simulink library "UAVdesign_net"  (Simulink 7.7)
settings: Solver=ode45  SolverMode=SingleTasking  StartTime=0.0  StopTime=10.0  RelTol=1e-3
undefined symbols (not defined in the file or in its folder): alpha_IERA_IELA_IELA, R_IERA_RA_RA
libraries: UAVdesign_net x75, simulink x13
(part 4 of 8)

== system UAVdesign_net/Subsystem Models/Helicopter Rotor/IERA to IELA ==
  T_IELA_IERA : Inport
  FM_I_IERA : Inport  Port=2
  FM_A_IERA : Inport  Port=3
  d_IERA : Inport  Port=4
  1D : Reshape
  Demux : Demux  Outputs=[6 6 3]
  Demux1 : Demux  Outputs=2
  Demux2 : Demux  Outputs=2
  Product : Product  Multiplication=Matrix(*)  RndMeth=Zero
  Signal Specification{,1..4} (5 alike) : SignalSpecification  Dimensions=3
  Vector Concatenate : Concatenate  NumInputs=5  Mode=Multidimensional array  ConcatenateDimension=2
  FM_I_IELA : Outport
  FM_A_IELA : Outport  Port=2
  d_IELA : Outport  Port=3
  wires:
  FM_A_IERA/1 -> Demux2/1
  Demux2/2 -> Signal Specification3/1
  Demux2/1 -> Signal Specification2/1
  Demux1/1 -> Signal Specification/1
  Demux1/2 -> Signal Specification1/1
  FM_I_IERA/1 -> Demux1/1
  d_IERA/1 -> Signal Specification4/1
  Demux/3 -> d_IELA/1
  Demux/2 -> FM_A_IELA/1
  Demux/1 -> FM_I_IELA/1
  1D/1 -> Demux/1
  Product/1 -> 1D/1
  Vector Concatenate/1 -> Product/2
  T_IELA_IERA/1 -> Product/1
  Signal Specification/1 -> Vector Concatenate/1
  Signal Specification1/1 -> Vector Concatenate/2
  Signal Specification2/1 -> Vector Concatenate/3
  Signal Specification3/1 -> Vector Concatenate/4
  Signal Specification4/1 -> Vector Concatenate/5

== system UAVdesign_net/Subsystem Models/Helicopter Rotor/Rotor Model (IERA) ==
  Parameters : Inport  OutDataTypeStr=Bus: RotorParameters
  Environment : Inport  Port=2  OutDataTypeStr=Bus: Environment
  V_I : Inport  Port=3  PortDimensions=3
  omega_I : Inport  Port=4  PortDimensions=3
  V_dot_I : Inport  Port=5  PortDimensions=3
  omega_dot_I : Inport  Port=6  PortDimensions=3
  V_A : Inport  Port=7  PortDimensions=3
  omega_A : Inport  Port=8  PortDimensions=3
  omega_rotor : Inport  Port=9  PortDimensions=1
  omega_dot_rotor : Inport  Port=10  PortDimensions=1
  controls : Inport  Port=11  PortDimensions=3
  flap : Inport  Port=12  PortDimensions=3
  bt (k-1) : Inport  Port=13  PortDimensions=1
  eps0 (k-1) : Inport  Port=14  PortDimensions=1
  Ch Sign Lift : Gain  Gain=[-1 1]
  IERA to WM : Subsystem
      mask Display:
      | port_label('input', 1, 'T_{WM-IERA}', 'texmode', 'on')
      | port_label('input', 2, 'V_{I|IERA}', 'texmode', 'on')
      | port_label('input', 3, '\omega_{I|IERA}', 'texmode', 'on')
      | port_label('input', 4, 'V^\bullet_{I|IERA}', 'texmode', 'on')
      | port_label('input', 5, '\omega^\bullet_{I|IERA}', 'texmode', 'on')
      | port_label('input', 6, 'V_{A|IERA}', 'texmode', 'on')
      | port_label('input', 7, '\omega_{A|IERA}', 'texmode', 'on')
      | port_label('input', 8, 'controls_{IERA}', 'texmode', 'on')
      | port_label('input', 9, 'flap_{IERA}', 'texmode', 'on')
      | 
      | port_label('output', 1, 'V_{I|WM}', 'texmode', 'on')
      | port_label('output', 2, '\omega_{I|WM}', 'texmode', 'on')
      | port_label('output', 3, 'V^\bullet_{I|WM}', 'texmode', 'on')
      | port_label('output', 4, '\omega^\bullet_{I|WM}', 'texmode', 'on')
      | port_label('output', 5, 'V_{A|WM}', 'texmode', 'on')
      | port_label('output', 6, '\omega_{A|WM}', 'texmode', 'on')
      | port_label('output', 7, 'controls_{WM}', 'texmode', 'on')
      | port_label('output', 8, 'flap_{WM}', 'texmode', 'on')
  Rotor Flapping : Subsystem
      mask Display:
      | port_label('input', 1, 'Parameters', 'texmode', 'on')
      | port_label('input', 2, 'Environment', 'texmode', 'on')
      | port_label('input', 3, 'V_{I|WM}', 'texmode', 'on')
      | port_label('input', 4, '\omega_{I|WM}', 'texmode', 'on')
      | port_label('input', 5, 'V^\bullet_{I|WM}', 'texmode', 'on')
      | port_label('input', 6, '\omega^\bullet_{I|WM}', 'texmode', 'on')
      | port_label('input', 7, 'V_{A|WM}', 'texmode', 'on')
      | port_label('input', 8, '\omega_{A|WM}', 'texmode', 'on')
      | port_label('input', 9, 'flap_{WM}', 'texmode', 'on')
      | port_label('input', 10, 'cz', 'texmode', 'on')
      | port_label('input', 11, 'controls_{WM}', 'texmode', 'on')
      | port_label('input', 12, '\Omega_{rotor}', 'texmode', 'on')
      | 
      | port_label('output', 1, 'flap^\bullet_{WM}', 'texmode', 'on')
      | port_label('output', 2, 'flap-static_{WM}', 'texmode', 'on')
  Rotor Forces and Moments : Subsystem
      mask Display:
      | port_label('input', 1, 'Parameters', 'texmode', 'on')
      | port_label('input', 2, 'Environment', 'texmode', 'on')
      | port_label('input', 3, 'V_{A|WM}', 'texmode', 'on')
      | port_label('input', 4, '\omega_{A|WM}', 'texmode', 'on')
      | port_label('input', 5, '\omega^\bullet_{I|WM}', 'texmode', 'on')
      | port_label('input', 6, 'flap_{WM}', 'texmode', 'on')
      | port_label('input', 7, 'cz', 'texmode', 'on')
      | port_label('input', 8, 'controls_{WM}', 'texmode', 'on')
      | port_label('input', 9, '\Omega_{rotor}', 'texmode', 'on')
      | port_label('input', 10, '\Omega^\bullet_{rotor}', 'texmode', 'on')
      | 
      | port_label('output', 1, 'FM_{A}', 'texmode', 'on')
      | port_label('output', 2, 'FM_{I}', 'texmode', 'on')
  Rotor Self-Influence : Subsystem
      mask Display:
      | port_label('input', 1, 'Parameters', 'texmode', 'on')
      | port_label('input', 2, 'Environment', 'texmode', 'on')
      | port_label('input', 3, 'V_{A|IERA}', 'texmode', 'on')
      | port_label('input', 4, '\omega_{A|IERA}', 'texmode', 'on')
      | port_label('input', 5, 'FM_{A|IERA}', 'texmode', 'on')
      | 
      | port_label('output', 1, 'd_{k|IERA}', 'texmode', 'on')
  Rotor Wash Iteration : Subsystem
      mask Display:
      | port_label('input', 1, 'Parameters', 'texmode', 'on')
      | port_label('input', 2, 'V_{I|WM}', 'texmode', 'on')
      | port_label('input', 3, 'V_{A k-1|WM}', 'texmode', 'on')
      | port_label('input', 4, '\omega_{A|WM}', 'texmode', 'on')
      | port_label('input', 5, 'bt_{k-1}', 'texmode', 'on')
      | port_label('input', 6, 'eps0_{k-1}', 'texmode', 'on')
      | port_label('input', 7, 'controls_{WM}', 'texmode', 'on')
      | port_label('input', 8, '\Omega_{rotor}', 'texmode', 'on')
      | 
      | port_label('output', 1, 'V_{A k|WM}', 'texmode', 'on')
      | port_label('output', 2, 'cz_{k|WM}', 'texmode', 'on')
      | port_label('output', 3, 'bt_{k}', 'texmode', 'on')
      | port_label('output', 4, 'eps_{k}', 'texmode', 'on')
  T Q : Selector  InputPortWidth=6  IndexOptions=Index vector (dialog)  Indices=[3 6]  OutputSizes=1
  WM to IERA : Subsystem
      mask Display:
      | port_label('input', 1, 'T_{IERA-WM}', 'texmode', 'on')
      | port_label('input', 2, 'FM_{A|WM}', 'texmode', 'on')
      | port_label('input', 3, 'FM_{I|WM}', 'texmode', 'on')
      | port_label('input', 4, 'V_{A k|WM}', 'texmode', 'on')
      | port_label('input', 5, 'flap^\bullet_{WM}', 'texmode', 'on')
      | port_label('input', 6, 'flap_{WM}', 'texmode', 'on')
      | 
      | port_label('output', 1, 'FM_{A|IERA}', 'texmode', 'on')
      | port_label('output', 2, 'FM_{I|IERA}', 'texmode', 'on')
      | port_label('output', 3, 'V_{A k|IERA}', 'texmode', 'on')
      | port_label('output', 4, 'flap^\bullet_{IERA}', 'texmode', 'on')
      | port_label('output', 5, 'flap_{IERA}', 'texmode', 'on')
  Wind-Mast Orientation : Subsystem
      mask Display:
      | port_label('input', 1, 'V_{A|IERA}', 'texmode', 'on')
      | port_label('output', 1, 'T_{WM-IERA}', 'texmode', 'on')
      | port_label('output', 2, 'T_{IERA-WM}', 'texmode', 'on')
  FM_I : Outport  PortDimensions=6
  FM_A : Outport  Port=2  PortDimensions=6
  d (k) : Outport  Port=3  PortDimensions=3
  flap_dot : Outport  Port=4  PortDimensions=3
  flap (k) : Outport  Port=5  PortDimensions=3
  bt (k) : Outport  Port=6  PortDimensions=1
  eps0 (k) : Outport  Port=7  PortDimensions=1
  TQ : Outport  Port=8  PortDimensions=2
  wires:
  eps0 (k-1)/1 -> Rotor Wash Iteration/6(eps0 (k-1))
  bt (k-1)/1 -> Rotor Wash Iteration/5(bt (k-1))
  Rotor Wash Iteration/4(eps0 (k)) -> eps0 (k)/1
  Rotor Wash Iteration/3(bt (k)) -> bt (k)/1
  WM to IERA/5(flap_IERA) -> flap (k)/1
  WM to IERA/4(flap_dot_IERA) -> flap_dot/1
  WM to IERA/1(FM_A_IERA) -> FM_A/1, Rotor Self-Influence/5(FM_A)
  WM to IERA/2(FM_I_IERA) -> FM_I/1
  Rotor Flapping/2(flap_static) -> WM to IERA/6(flap_WM)
  Rotor Flapping/1(flap_dot) -> WM to IERA/5(flap_dot_WM)
  Rotor Forces and Moments/2(FM_I) -> WM to IERA/3(FM_I_WM)
  Rotor Forces and Moments/1(FM_A) -> WM to IERA/2(FM_A_WM), T Q/1
  Wind-Mast Orientation/2(T_IERA_WM) -> WM to IERA/1(T_IERA_WM)
  omega_dot_rotor/1 -> Rotor Forces and Moments/10(omega_dot_rotor)
  omega_rotor/1 -> Rotor Forces and Moments/9(omega_rotor), Rotor Wash Iteration/8(omega_rotor), Rotor Flapping/12(omega)
  IERA to WM/8(flap_WM) -> Rotor Forces and Moments/6(flap), Rotor Flapping/9(flap)
  IERA to WM/7(controls_WM) -> Rotor Wash Iteration/7(controls), Rotor Flapping/11(controls), Rotor Forces and Moments/8(controls)
  Rotor Wash Iteration/2(cz (k)) -> Rotor Flapping/10(cz), Rotor Forces and Moments/7(cz)
  IERA to WM/1(V_I_WM) -> Rotor Flapping/3(V_I), Rotor Wash Iteration/2(V_I)
  IERA to WM/2(omega_I_WM) -> Rotor Flapping/4(omega_I)
  IERA to WM/3(V_dot_I_WM) -> Rotor Flapping/5(V_dot_I)
  IERA to WM/4(omega_dot_I_WM) -> Rotor Flapping/6(omega_dot_I), Rotor Forces and Moments/5(omega_dot_I)
  IERA to WM/6(omega_A_WM) -> Rotor Wash Iteration/4(omega_A), Rotor Flapping/8(omega_A), Rotor Forces and Moments/4(omega_A)
  Environment/1 -> Rotor Forces and Moments/2(Environment), Rotor Flapping/2(Environment), Rotor Self-Influence/2(Environment)
  Parameters/1 -> Rotor Forces and Moments/1(Parameters), Rotor Flapping/1(Parameters), Rotor Wash Iteration/1(Parameters), Rotor Self-Influence/1(Parameters)
  flap/1 -> IERA to WM/9(flap_IERA)
  omega_I/1 -> IERA to WM/3(omega_I_IERA)
  controls/1 -> IERA to WM/8(controls_IERA)
  Wind-Mast Orientation/1(T_WM_IERA) -> IERA to WM/1(T_WM_IERA)
  omega_A/1 -> IERA to WM/7(omega_A_IERA), Rotor Self-Influence/4(omega_A)
  V_A/1 -> Wind-Mast Orientation/1(V_A), IERA to WM/6(V_A_IERA)
  omega_dot_I/1 -> IERA to WM/5(omega_dot_I_IERA)
  V_dot_I/1 -> IERA to WM/4(V_dot_I_IERA)
  V_I/1 -> IERA to WM/2(V_I_IERA)
  IERA to WM/5(V_A_WM) -> Rotor Wash Iteration/3(V_A (k-1))
  Rotor Wash Iteration/1(V_A (k)) -> Rotor Forces and Moments/3(V_A), Rotor Flapping/7(V_A), WM to IERA/4(d_WM)
  WM to IERA/3(d_IERA) -> Rotor Self-Influence/3(V_A)
  Rotor Self-Influence/1(d (k)) -> d (k)/1
  T Q/1 -> Ch Sign Lift/1
  Ch Sign Lift/1 -> TQ/1

== system UAVdesign_net/Subsystem Models/Helicopter Rotor/Transpose ==
  In : Inport
  Permute Dimensions : PermuteDimensions
  Out : Outport
  wires:
  In/1 -> Permute Dimensions/1
  Permute Dimensions/1 -> Out/1

== system UAVdesign_net/Subsystem Models/Propeller/CG to IELA ==
  R_IELA-B|B : Inport
  V_B-E|B : Inport  Port=2
  omega_B_E|B : Inport  Port=3
  3x3 Cross Product : UAVdesign_net/Utilities/Math/3x3 Cross Product  SystemSampleTime=-1
  Sum : Sum  Inputs=++|
  V_IELA-E|IELA : Outport
  omega_IELA-E|IELA : Outport  Port=2
  wires:
  omega_B_E|B/1 -> 3x3 Cross Product/1, omega_IELA-E|IELA/1
  R_IELA-B|B/1 -> 3x3 Cross Product/2
  3x3 Cross Product/1 -> Sum/2
  V_B-E|B/1 -> Sum/1
  Sum/1 -> V_IELA-E|IELA/1

== system UAVdesign_net/Subsystem Models/Propeller/Direction of Rotation ==
  Parameters : Inport
  V_B-E|B_in : Inport  Port=2
  omega_B_E|B_in : Inport  Port=3
  V_W|B_in : Inport  Port=4
  omega_W|B_in : Inport  Port=5
  d|B_in : Inport  Port=6
  Bus Selector : BusSelector  OutputSignals=azsign
  Constant : Constant
  Mux : Mux  Inputs=3
  Mux1 : Mux  Inputs=3
  Product{,1..4} (5 alike) : Product  RndMeth=Zero
  Unary Minus : UnaryMinus
  V_B-E|B : Outport
  omega_B_E|B : Outport  Port=2
  V_W|B : Outport  Port=3
  omega_W|B : Outport  Port=4
  d|B : Outport  Port=5
  wires:
  Parameters/1 -> Bus Selector/1
  Bus Selector/1 -> Unary Minus/1  "<azsign>"
  Unary Minus/1 -> Mux/1, Mux/3, Mux1/2
  Constant/1 -> Mux/2, Mux1/1, Mux1/3
  V_B-E|B_in/1 -> Product/2
  Product/1 -> V_B-E|B/1
  Mux1/1 -> Product/1, Product3/1, Product4/1
  Mux/1 -> Product2/1, Product1/1
  omega_B_E|B_in/1 -> Product2/2
  Product2/1 -> omega_B_E|B/1
  Product3/1 -> V_W|B/1
  Product1/1 -> omega_W|B/1
  Product4/1 -> d|B/1
  V_W|B_in/1 -> Product3/2
  omega_W|B_in/1 -> Product1/2
  d|B_in/1 -> Product4/2

== system UAVdesign_net/Subsystem Models/Propeller/Direction of Rotation 2 ==
  Parameters : Inport
  FM_IELA_in : Inport  Port=2
  d_IELA_in : Inport  Port=3
  Bus Selector : BusSelector  OutputSignals=azsign
  Constant : Constant
  Mux : Mux  Inputs=6
  Mux1 : Mux  Inputs=3
  Product : Product  RndMeth=Zero
  Product1 : Product  RndMeth=Zero
  Unary Minus : UnaryMinus
  FM_IELA : Outport
  d_IELA : Outport  Port=2
  wires:
  Product/1 -> FM_IELA/1
  FM_IELA_in/1 -> Product/2
  Bus Selector/1 -> Unary Minus/1  "<azsign>"
  Parameters/1 -> Bus Selector/1
  Unary Minus/1 -> Mux/2, Mux/4, Mux/6, Mux1/2
  Constant/1 -> Mux/1, Mux/3, Mux/5, Mux1/1, Mux1/3
  Mux/1 -> Product/1
  Mux1/1 -> Product1/1
  Product1/1 -> d_IELA/1
  d_IELA_in/1 -> Product1/2

== system UAVdesign_net/Subsystem Models/Propeller/IELA to CG ==
  R_IELA_B_B : Inport
  FM_IELA : Inport  Port=2
  3x3 Cross Product : UAVdesign_net/Utilities/Math/3x3 Cross Product  SystemSampleTime=-1
  Demux : Demux  Outputs=2
  Mux : Mux  Inputs=2
  Sum : Sum  Inputs=++|
  FM_B : Outport
  wires:
  FM_IELA/1 -> Demux/1
  Mux/1 -> FM_B/1
  Demux/1 -> Mux/1, 3x3 Cross Product/2
  R_IELA_B_B/1 -> 3x3 Cross Product/1
  Demux/2 -> Sum/2
  Sum/1 -> Mux/2
  3x3 Cross Product/1 -> Sum/1

== system UAVdesign_net/Subsystem Models/Propeller/IELA to IERA ==
  T_IERA_IELA : Inport
  V_I_IELA : Inport  Port=2
  omega_I_IELA : Inport  Port=3
  V_A_IELA : Inport  Port=4
  omega_A_IELA : Inport  Port=5
  1D : Reshape
  Demux : Demux
  Product : Product  Multiplication=Matrix(*)  RndMeth=Zero
  Vector Concatenate : Concatenate  NumInputs=4  Mode=Multidimensional array  ConcatenateDimension=2
  V_I_IERA : Outport
  omega_I_IERA : Outport  Port=2
  V_A_IERA : Outport  Port=3
  omega_A_IERA : Outport  Port=4
  wires:
  T_IERA_IELA/1 -> Product/1
  V_I_IELA/1 -> Vector Concatenate/1
  omega_I_IELA/1 -> Vector Concatenate/2
  Vector Concatenate/1 -> Product/2
  Product/1 -> 1D/1
  1D/1 -> Demux/1
  Demux/1 -> V_I_IERA/1
  Demux/2 -> omega_I_IERA/1
  Demux/3 -> V_A_IERA/1
  Demux/4 -> omega_A_IERA/1
  V_A_IELA/1 -> Vector Concatenate/3
  omega_A_IELA/1 -> Vector Concatenate/4

== system UAVdesign_net/Subsystem Models/Propeller/IERA to IELA ==
  T_IELA_IERA : Inport
  FM_IERA : Inport  Port=2
  d_IERA : Inport  Port=3
  1D : Reshape
  Demux : Demux  Outputs=[6 3]
  Demux1 : Demux  Outputs=2
  Product : Product  Multiplication=Matrix(*)  RndMeth=Zero
  Signal Specification : SignalSpecification  Dimensions=3
  Signal Specification1 : SignalSpecification  Dimensions=3
  Signal Specification4 : SignalSpecification  Dimensions=3
  Vector Concatenate : Concatenate  NumInputs=3  Mode=Multidimensional array  ConcatenateDimension=2
  FM_IELA : Outport
  d_IELA : Outport  Port=2
  wires:
  Signal Specification4/1 -> Vector Concatenate/3
  Signal Specification1/1 -> Vector Concatenate/2
  Signal Specification/1 -> Vector Concatenate/1
  T_IELA_IERA/1 -> Product/1
  Vector Concatenate/1 -> Product/2
  Product/1 -> 1D/1
  1D/1 -> Demux/1
  Demux/1 -> FM_IELA/1
  d_IERA/1 -> Signal Specification4/1
  FM_IERA/1 -> Demux1/1
  Demux1/2 -> Signal Specification1/1
  Demux1/1 -> Signal Specification/1
  Demux/2 -> d_IELA/1

== system UAVdesign_net/Subsystem Models/Propeller/Rotor Forces and Moments (Inertial) ==
  Parameters : Inport
  FM_A_IERA : Inport  Port=2
  omega_I : Inport  Port=3
  omega_rotor : Inport  Port=4
  torque_motor : Inport  Port=5
  Rotor Forces and Moments (IERA) : Stateflow chart  TreatAsAtomicUnit=on
  FM_total : Outport  PortDimensions=6
  wires:
  FM_A_IERA/1 -> Rotor Forces and Moments (IERA)/5(FM_A)
  omega_I/1 -> Rotor Forces and Moments (IERA)/2(omi)
  Rotor Forces and Moments (IERA)/1(FM_total) -> FM_total/1
  Parameters/1 -> Rotor Forces and Moments (IERA)/1(Parameters)
  omega_rotor/1 -> Rotor Forces and Moments (IERA)/3(omega)
  torque_motor/1 -> Rotor Forces and Moments (IERA)/4(tau_motor)

== system UAVdesign_net/Subsystem Models/Propeller/Rotor Model (IERA) ==
  Parameters : Inport
  Environment : Inport  Port=2
  V_I : Inport  Port=3  PortDimensions=3
  omega_I : Inport  Port=4  PortDimensions=3
  V_A : Inport  Port=5  PortDimensions=3
  omega_A : Inport  Port=6  PortDimensions=3
  omega_rotor : Inport  Port=7  PortDimensions=1
  controls : Inport  Port=8  PortDimensions=1
  bt (k-1) : Inport  Port=9  PortDimensions=1
  eps0 (k-1) : Inport  Port=10  PortDimensions=1
  Ch Sign Lift : Gain  Gain=[-1 1]
  IERA to WM : Subsystem
      mask Display:
      | port_label('input', 1, 'T_{WM-IERA}', 'texmode', 'on')
      | port_label('input', 2, 'V_{I|IERA}', 'texmode', 'on')
      | port_label('input', 3, '\omega_{I|IERA}', 'texmode', 'on')
      | port_label('input', 4, 'V_{A|IERA}', 'texmode', 'on')
      | port_label('input', 5, '\omega_{A|IERA}', 'texmode', 'on')
      | 
      | port_label('output', 1, 'V_{I|WM}', 'texmode', 'on')
      | port_label('output', 2, '\omega_{I|WM}', 'texmode', 'on')
      | port_label('output', 3, 'V_{A|WM}', 'texmode', 'on')
      | port_label('output', 4, '\omega_{A|WM}', 'texmode', 'on')
  Rotor Forces and Moments (Aero) : Subsystem
      mask Display:
      | port_label('input', 1, 'Parameters', 'texmode', 'on')
      | port_label('input', 2, 'Environment', 'texmode', 'on')
      | port_label('input', 3, 'V_{A|WM}', 'texmode', 'on')
      | port_label('input', 4, '\omega_{A|WM}', 'texmode', 'on')
      | port_label('input', 5, 'cz', 'texmode', 'on')
      | port_label('input', 6, 'controls_{WM}', 'texmode', 'on')
      | port_label('input', 7, '\Omega_{rotor}', 'texmode', 'on')
      | 
      | port_label('output', 1, 'FM_{A}', 'texmode', 'on')
  Rotor Self-Influence : Subsystem
      mask Display:
      | port_label('input', 1, 'Parameters', 'texmode', 'on')
      | port_label('input', 2, 'Environment', 'texmode', 'on')
      | port_label('input', 3, 'V_{A|IERA}', 'texmode', 'on')
      | port_label('input', 4, '\omega_{A|IERA}', 'texmode', 'on')
      | port_label('input', 5, 'FM_{A|IERA}', 'texmode', 'on')
      | 
      | port_label('output', 1, 'd_{k|IERA}', 'texmode', 'on')
  Rotor Wash Iteration : Subsystem
      mask Display:
      | port_label('input', 1, 'Parameters', 'texmode', 'on')
      | port_label('input', 2, 'V_{I|WM}', 'texmode', 'on')
      | port_label('input', 3, 'V_{A k-1|WM}', 'texmode', 'on')
      | port_label('input', 4, '\omega_{A|WM}', 'texmode', 'on')
      | port_label('input', 5, 'bt_{k-1}', 'texmode', 'on')
      | port_label('input', 6, 'eps0_{k-1}', 'texmode', 'on')
      | port_label('input', 7, 'controls_{WM}', 'texmode', 'on')
      | port_label('input', 8, '\Omega_{rotor}', 'texmode', 'on')
      | 
      | port_label('output', 1, 'V_{A k|WM}', 'texmode', 'on')
      | port_label('output', 2, 'cz_{k|WM}', 'texmode', 'on')
      | port_label('output', 3, 'bt_{k}', 'texmode', 'on')
      | port_label('output', 4, 'eps_{k}', 'texmode', 'on')
  T Q : Selector  InputPortWidth=6  IndexOptions=Index vector (dialog)  Indices=[3 6]  OutputSizes=1
  Terminator : Terminator
  WM to IERA : Subsystem
      mask Display:
      | port_label('input', 1, 'T_{IERA-WM}', 'texmode', 'on')
      | port_label('input', 2, 'FM_{A|WM}', 'texmode', 'on')
      | port_label('input', 3, 'V_{A k|WM}', 'texmode', 'on')
      | 
      | port_label('output', 1, 'FM_{A|IERA}', 'texmode', 'on')
      | port_label('output', 2, 'V_{A k|IERA}', 'texmode', 'on')
  Wind-Mast Orientation : Subsystem
      mask Display:
      | port_label('input', 1, 'V_{A|IERA}', 'texmode', 'on')
      | port_label('output', 1, 'T_{WM-IERA}', 'texmode', 'on')
      | port_label('output', 2, 'T_{IERA-WM}', 'texmode', 'on')
  FM_A : Outport  PortDimensions=6
  d (k) : Outport  Port=2  PortDimensions=3
  bt (k) : Outport  Port=3  PortDimensions=1
  eps0 (k) : Outport  Port=4  PortDimensions=1
  TQ : Outport  Port=5  PortDimensions=2
  wires:
  Ch Sign Lift/1 -> TQ/1
  T Q/1 -> Ch Sign Lift/1
  Rotor Self-Influence/1(d (k)) -> d (k)/1
  WM to IERA/2(d_IERA) -> Rotor Self-Influence/3(V_A)
  Rotor Wash Iteration/1(V_A (k)) -> WM to IERA/3(d_WM), Rotor Forces and Moments (Aero)/3(V_A)
  IERA to WM/3(V_A_WM) -> Rotor Wash Iteration/3(V_A (k-1))
  V_I/1 -> IERA to WM/2(V_I_IERA)
  V_A/1 -> IERA to WM/4(V_A_IERA), Wind-Mast Orientation/1(V_A)
  omega_A/1 -> Rotor Self-Influence/4(omega_A), IERA to WM/5(omega_A_IERA)
  Wind-Mast Orientation/1(T_WM_IERA) -> IERA to WM/1(T_WM_IERA)
  omega_I/1 -> IERA to WM/3(omega_I_IERA)
  Parameters/1 -> Rotor Forces and Moments (Aero)/1(Parameters), Rotor Wash Iteration/1(Parameters), Rotor Self-Influence/1(Parameters)
  Environment/1 -> Rotor Forces and Moments (Aero)/2(Environment), Rotor Self-Influence/2(Environment)
  IERA to WM/4(omega_A_WM) -> Rotor Forces and Moments (Aero)/4(omega_A), Rotor Wash Iteration/4(omega_A)
  IERA to WM/1(V_I_WM) -> Rotor Wash Iteration/2(V_I)
  Rotor Wash Iteration/2(cz (k)) -> Rotor Forces and Moments (Aero)/5(cz)
  omega_rotor/1 -> Rotor Wash Iteration/8(omega_rotor), Rotor Forces and Moments (Aero)/7(omega_rotor)
  Wind-Mast Orientation/2(T_IERA_WM) -> WM to IERA/1(T_IERA_WM)
  Rotor Forces and Moments (Aero)/1(FM_A) -> T Q/1, WM to IERA/2(FM_A_WM)
  WM to IERA/1(FM_A_IERA) -> FM_A/1, Rotor Self-Influence/5(FM_A)
  Rotor Wash Iteration/3(bt (k)) -> bt (k)/1
  Rotor Wash Iteration/4(eps0 (k)) -> eps0 (k)/1
  bt (k-1)/1 -> Rotor Wash Iteration/5(bt (k-1))
  eps0 (k-1)/1 -> Rotor Wash Iteration/6(eps0 (k-1))
  controls/1 -> Rotor Forces and Moments (Aero)/6(controls), Rotor Wash Iteration/7(controls)
  IERA to WM/2(omega_I_WM) -> Terminator/1

== system UAVdesign_net/Subsystem Models/Propeller/Transpose ==
  In : Inport
  Permute Dimensions : PermuteDimensions
  Out : Outport
  wires:
  Permute Dimensions/1 -> Out/1
  In/1 -> Permute Dimensions/1

== system UAVdesign_net/Subsystem Models/Propeller Rotation Dynamics/Direction of Rotation ==
  Parameters : Inport
  omega_B_E|B_in : Inport  Port=2
  omega_dot_B_E|B_in : Inport  Port=3
  Bus Selector : BusSelector  OutputSignals=azsign
  Constant : Constant
  Mux : Mux  Inputs=3
  Product1 : Product  RndMeth=Zero
  Product2 : Product  RndMeth=Zero
  Unary Minus : simulink/Math Operations/Unary Minus  DoSatur=off
  omega_B_E|B : Outport
  omega_dot_B_E|B : Outport  Port=2
  wires:
  Product2/1 -> omega_B_E|B/1
  omega_B_E|B_in/1 -> Product2/2
  Mux/1 -> Product2/1, Product1/1
  Constant/1 -> Mux/2
  Unary Minus/1 -> Mux/1, Mux/3
  Bus Selector/1 -> Unary Minus/1  "<azsign>"
  Parameters/1 -> Bus Selector/1
  Product1/1 -> omega_dot_B_E|B/1
  omega_dot_B_E|B_in/1 -> Product1/2

== system UAVdesign_net/Subsystem Models/Propeller Rotation Dynamics/IELA to IERA ==
  T_IERA_IELA : Inport
  omega_I_IELA : Inport  Port=2
  omega_dot_I_IELA : Inport  Port=3
  1D : Reshape
  Demux : Demux  Outputs=2
  Product : Product  Multiplication=Matrix(*)  RndMeth=Zero
  Vector Concatenate : Concatenate  Mode=Multidimensional array  ConcatenateDimension=2
  omega_I_IERA : Outport
  omega_dot_I_IERA : Outport  Port=2
  wires:
  1D/1 -> Demux/1
  Product/1 -> 1D/1
  Vector Concatenate/1 -> Product/2
  T_IERA_IELA/1 -> Product/1
  omega_I_IELA/1 -> Vector Concatenate/1
  omega_dot_I_IELA/1 -> Vector Concatenate/2
  Demux/2 -> omega_dot_I_IERA/1
  Demux/1 -> omega_I_IERA/1

== system UAVdesign_net/Subsystem Models/QuadRotor Parameters/Fuse Parameters ==
  In : Inport
  Bus Creator : BusCreator  Inputs=7  OutDataTypeStr=Bus: FuselageParameters  NonVirtualBus=on
  Demux : Demux  Outputs=17
  Vector Concatenate{,1..4} (5 alike) : Concatenate  NumInputs=3  Mode=Vector
  Parameters : Outport  OutDataTypeStr=Bus: FuselageParameters
  wires:
  Demux/1 -> Bus Creator/1  "carea"
  Bus Creator/1 -> Parameters/1
  In/1 -> Demux/1
  Demux/2 -> Bus Creator/2  "clen"
  Demux/3 -> Vector Concatenate/1
  Demux/4 -> Vector Concatenate/2
  Demux/5 -> Vector Concatenate/3
  Vector Concatenate/1 -> Bus Creator/3  "cx"
  Demux/6 -> Vector Concatenate1/1
  Demux/7 -> Vector Concatenate1/2
  Demux/8 -> Vector Concatenate1/3
  Vector Concatenate1/1 -> Bus Creator/4  "cy"
  Demux/9 -> Vector Concatenate2/1
  Demux/10 -> Vector Concatenate2/2
  Demux/11 -> Vector Concatenate2/3
  Vector Concatenate2/1 -> Bus Creator/5  "cz"
  Demux/12 -> Vector Concatenate3/1
  Demux/13 -> Vector Concatenate3/2
  Demux/14 -> Vector Concatenate3/3
  Demux/15 -> Vector Concatenate4/1
  Demux/16 -> Vector Concatenate4/2
  Demux/17 -> Vector Concatenate4/3
  Vector Concatenate3/1 -> Bus Creator/6  "cm"
  Vector Concatenate4/1 -> Bus Creator/7  "cn"

== system UAVdesign_net/Subsystem Models/QuadRotor Parameters/Motor Parameters ==
  In : Inport
  Bus Creator1 : BusCreator  Inputs=7  NonVirtualBus=on
  Data Type Conversion2 : DataTypeConversion  OutDataTypeStr=uint32  RndMeth=Nearest
  Demux1 : Demux  Outputs=7
  Parameters : Outport
  wires:
  In/1 -> Demux1/1
  Bus Creator1/1 -> Parameters/1
  Demux1/1 -> Bus Creator1/1  "R"
  Demux1/2 -> Bus Creator1/2  "L"
  Demux1/3 -> Bus Creator1/3  "Kv"
  Demux1/4 -> Bus Creator1/4  "Kt"
  Demux1/5 -> Data Type Conversion2/1
  Data Type Conversion2/1 -> Bus Creator1/5  "poles"
  Demux1/6 -> Bus Creator1/6  "In"
  Demux1/7 -> Bus Creator1/7  "Ngear"

== system UAVdesign_net/Subsystem Models/QuadRotor Parameters/Rotor Parameters ==
  In : Inport
  Bus Creator1 : BusCreator  Inputs=14  NonVirtualBus=on
  Data Type Conversion1 : DataTypeConversion  OutDataTypeStr=uint32  RndMeth=Nearest
  Data Type Conversion2 : DataTypeConversion  OutDataTypeStr=uint32  RndMeth=Nearest
  Demux1 : Demux  Outputs=16
  Gain1 : Gain  Gain=pi/180
  Gain3 : Gain  Gain=pi/180
  Vector Concatenate : Concatenate  NumInputs=3  Mode=Vector
  Parameters : Outport
  wires:
  Demux1/15 -> Bus Creator1/13  "azsign"
  Demux1/14 -> Bus Creator1/12  "mbar"
  Demux1/13 -> Bus Creator1/11  "iflap"
  Demux1/9 -> Bus Creator1/7  "btmax"
  Demux1/1 -> Bus Creator1/1  "a0"
  Bus Creator1/1 -> Parameters/1
  Demux1/4 -> Vector Concatenate/3
  Demux1/3 -> Vector Concatenate/2
  Demux1/2 -> Vector Concatenate/1
  In/1 -> Demux1/1
  Data Type Conversion1/1 -> Bus Creator1/3  "nb"
  Demux1/5 -> Data Type Conversion1/1
  Demux1/6 -> Bus Creator1/4  "radius"
  Demux1/7 -> Bus Creator1/5  "chord"
  Demux1/8 -> Bus Creator1/6  "btmin"
  Demux1/12 -> Gain3/1
  Demux1/10 -> Bus Creator1/8  "btq"
  Demux1/11 -> Gain1/1  "theta"
  Gain1/1 -> Bus Creator1/9  "theta"
  Vector Concatenate/1 -> Bus Creator1/2  "del0_2"
  Gain3/1 -> Bus Creator1/10  "twist"
  Demux1/16 -> Data Type Conversion2/1
  Data Type Conversion2/1 -> Bus Creator1/14  "flags"

== system UAVdesign_net/Subsystem Models/Wing/CG to IELA ==
  R_IELA-B|B : Inport
  V_B-E|B : Inport  Port=2
  omega_B_E|B : Inport  Port=3
  3x3 Cross Product : UAVdesign_net/Utilities/Math/3x3 Cross Product  SystemSampleTime=-1
  Sum : Sum  Inputs=++|
  V_IELA-E|IELA : Outport
  omega_IELA-E|IELA : Outport  Port=2
  wires:
  Sum/1 -> V_IELA-E|IELA/1
  V_B-E|B/1 -> Sum/1
  3x3 Cross Product/1 -> Sum/2
  R_IELA-B|B/1 -> 3x3 Cross Product/2
  omega_B_E|B/1 -> omega_IELA-E|IELA/1, 3x3 Cross Product/1

== system UAVdesign_net/Subsystem Models/Wing/IELA to CG ==
  R_IELA_B_B : Inport
  FM_IELA : Inport  Port=2
  3x3 Cross Product : UAVdesign_net/Utilities/Math/3x3 Cross Product  SystemSampleTime=-1
  Demux : Demux  Outputs=2
  Mux : Mux  Inputs=2
  Sum : Sum  Inputs=++|
  FM_B : Outport
  wires:
  3x3 Cross Product/1 -> Sum/1
  Sum/1 -> Mux/2
  Demux/2 -> Sum/2
  R_IELA_B_B/1 -> 3x3 Cross Product/1
  Demux/1 -> 3x3 Cross Product/2, Mux/1
  Mux/1 -> FM_B/1
  FM_IELA/1 -> Demux/1

== system UAVdesign_net/Subsystem Models/Wing/IELA to IERA ==
  T_IERA_IELA : Inport
  V_A_IELA : Inport  Port=2
  omega_A_IELA : Inport  Port=3
  V_W_IELA : Inport  Port=4
  omega_W_IELA : Inport  Port=5
  1D : Reshape
  Demux : Demux
  Product : Product  Multiplication=Matrix(*)  RndMeth=Zero
  Vector Concatenate : Concatenate  NumInputs=4  Mode=Multidimensional array  ConcatenateDimension=2
  V_A_IERA : Outport
  omega_A_IERA : Outport  Port=2
  V_W_IERA : Outport  Port=3
  omega_W_IERA : Outport  Port=4
  wires:
  omega_W_IELA/1 -> Vector Concatenate/4
  V_W_IELA/1 -> Vector Concatenate/3
  Demux/4 -> omega_W_IERA/1
  Demux/3 -> V_W_IERA/1
  Demux/2 -> omega_A_IERA/1
  Demux/1 -> V_A_IERA/1
  1D/1 -> Demux/1
  Product/1 -> 1D/1
  Vector Concatenate/1 -> Product/2
  omega_A_IELA/1 -> Vector Concatenate/2
  V_A_IELA/1 -> Vector Concatenate/1
  T_IERA_IELA/1 -> Product/1

== system UAVdesign_net/Subsystem Models/Wing/IERA to IELA ==
  T_IELA_IERA : Inport
  FM_I_IERA : Inport  Port=2
  FM_A_IERA : Inport  Port=3
  d_IERA : Inport  Port=4
  1D : Reshape
  Demux : Demux  Outputs=[6 6 3]
  Demux1 : Demux  Outputs=2
  Demux2 : Demux  Outputs=2
  Product : Product  Multiplication=Matrix(*)  RndMeth=Zero
  Signal Specification{,1..4} (5 alike) : SignalSpecification  Dimensions=3
  Vector Concatenate : Concatenate  NumInputs=5  Mode=Multidimensional array  ConcatenateDimension=2
  FM_I_IELA : Outport
  FM_A_IELA : Outport  Port=2
  d_IELA : Outport  Port=3
  wires:
  FM_A_IERA/1 -> Demux2/1
  Demux2/2 -> Signal Specification3/1
  Demux2/1 -> Signal Specification2/1
  Demux1/1 -> Signal Specification/1
  Demux1/2 -> Signal Specification1/1
  FM_I_IERA/1 -> Demux1/1
  d_IERA/1 -> Signal Specification4/1
  Demux/3 -> d_IELA/1
  Demux/2 -> FM_A_IELA/1
  Demux/1 -> FM_I_IELA/1
  1D/1 -> Demux/1
  Product/1 -> 1D/1
  Vector Concatenate/1 -> Product/2
  T_IELA_IERA/1 -> Product/1
  Signal Specification/1 -> Vector Concatenate/1
  Signal Specification1/1 -> Vector Concatenate/2
  Signal Specification2/1 -> Vector Concatenate/3
  Signal Specification3/1 -> Vector Concatenate/4
  Signal Specification4/1 -> Vector Concatenate/5

== system UAVdesign_net/Subsystem Models/Wing/Transpose ==
  In : Inport
  Permute Dimensions : PermuteDimensions
  Out : Outport
  wires:
  In/1 -> Permute Dimensions/1
  Permute Dimensions/1 -> Out/1

== system UAVdesign_net/Subsystem Models/Wing/Wing Model (IERA) ==
  Parameters : Inport  OutDataTypeStr=Bus: FinParameters
  Environment : Inport  Port=2  OutDataTypeStr=Bus: Environment
  V_A : Inport  Port=3
  omega_A : Inport  Port=4
  V_W : Inport  Port=5
  omega_W : Inport  Port=6
  control : Inport  Port=7
  Bus Selector : BusSelector  OutputSignals=dihedral,incid,sweep
  Euler Rotation Matrix MAC to WRA (Half Wing) : UAVdesign_net/Utilities/Axes/Euler Rotation Matrix from Earth to Body  SystemSampleTime=-1
  Left : Constant  Value=-1
  Left Wing : Subsystem
      mask Display:
      | port_label('input', 1, 'Parameters', 'texmode', 'on')
      | port_label('input', 2, 'Environment', 'texmode', 'on')
      | port_label('input', 3, 'V_{A}', 'texmode', 'on')
      | port_label('input', 4, '\omega_{A}', 'texmode', 'on')
      | port_label('input', 5, 'T_{WRA-MAC}', 'texmode', 'on')
      | port_label('input', 6, 'T_{MAC-WRA}', 'texmode', 'on')
      | port_label('input', 7, 'Left/Right', 'texmode', 'on')
      | 
      | port_label('output', 1, 'FM_{A}', 'texmode', 'on')
  Mux : Mux  Inputs=3
  Right : Constant
  Right Wing : Subsystem
      mask Display:
      | port_label('input', 1, 'Parameters', 'texmode', 'on')
      | port_label('input', 2, 'Environment', 'texmode', 'on')
      | port_label('input', 3, 'V_{A}', 'texmode', 'on')
      | port_label('input', 4, '\omega_{A}', 'texmode', 'on')
      | port_label('input', 5, 'T_{WRA-MAC}', 'texmode', 'on')
      | port_label('input', 6, 'T_{MAC-WRA}', 'texmode', 'on')
      | port_label('input', 7, 'Left/Right', 'texmode', 'on')
      | 
      | port_label('output', 1, 'FM_{A}', 'texmode', 'on')
  Sum : Sum  Inputs=|++
  Sum1 : Sum  Inputs=|++
  Terminator : Terminator
  Terminator1 : Terminator
  Transpose : Subsystem
      mask Display: disp('A^T', 'texmode', 'on')
  Unary Minus : simulink/Math Operations/Unary Minus  DoSatur=off
  Wing Self-Influence : Subsystem
      mask Display:
      | port_label('input', 1, 'Parameters', 'texmode', 'on')
      | port_label('input', 2, 'Environment', 'texmode', 'on')
      | port_label('input', 3, 'V_{A|IERA}', 'texmode', 'on')
      | port_label('input', 4, '\omega_{A|IERA}', 'texmode', 'on')
      | port_label('input', 5, 'FM_{A|IERA}', 'texmode', 'on')
      | 
      | port_label('output', 1, 'd_{k|IERA}', 'texmode', 'on')
  Zero inertial : Constant  Value=[0 0 0 0 0 0]
  FM_I : Outport
  FM_A : Outport  Port=2
  d (k) : Outport  Port=3
  wires:
  Wing Self-Influence/1(d (k)) -> d (k)/1
  Left Wing/1(FM_A) -> Sum1/2
  Sum1/1 -> Wing Self-Influence/5(FM_A), FM_A/1
  Right Wing/1(FM_A) -> Sum1/1
  Left/1 -> Left Wing/7(Left/Right)
  Right/1 -> Right Wing/7(Left/Right)
  Zero inertial/1 -> FM_I/1
  omega_W/1 -> Terminator1/1
  V_W/1 -> Terminator/1
  omega_A/1 -> Wing Self-Influence/4(omega_A), Left Wing/4(omega_A), Right Wing/4(omega_A)
  V_A/1 -> Wing Self-Influence/3(V_A), Left Wing/3(V_A), Right Wing/3(V_A)
  control/1 -> Sum/2
  Sum/1 -> Mux/2
  Bus Selector/3 -> Mux/3  "<sweep>"
  Bus Selector/2 -> Sum/1  "<incid>"
  Bus Selector/1 -> Unary Minus/1  "<dihedral>"
  Unary Minus/1 -> Mux/1
  Mux/1 -> Euler Rotation Matrix MAC to WRA (Half Wing)/1
  Transpose/1(Out) -> Left Wing/6(T_MAC_WRA), Right Wing/6(T_MAC_WRA)
  Euler Rotation Matrix MAC to WRA (Half Wing)/1 -> Left Wing/5(T_WRA_MAC), Right Wing/5(T_WRA_MAC), Transpose/1(In)
  Environment/1 -> Wing Self-Influence/2(Environment), Left Wing/2(Environment), Right Wing/2(Environment)
  Parameters/1 -> Wing Self-Influence/1(Parameters), Left Wing/1(Parameters), Right Wing/1(Parameters), Bus Selector/1

== system UAVdesign_net/Utilities/Axes/Attitude Estimation ==
  V_e_1 : Inport  PortDimensions=3
  V_b_1 : Inport  Port=2  PortDimensions=3
  a1 : Inport  Port=3  PortDimensions=1
  V_e_2 : Inport  Port=4  PortDimensions=3
  V_b_2 : Inport  Port=5  PortDimensions=3
  a2 : Inport  Port=6  PortDimensions=1
  Embedded MATLAB Function : Stateflow chart  TreatAsAtomicUnit=on
  Mux : Mux  Inputs=2
  Vector Concatenate : Concatenate  Mode=Multidimensional array  ConcatenateDimension=2
  Vector Concatenate1 : Concatenate  Mode=Multidimensional array  ConcatenateDimension=2
  q_be_opt : Outport
  wires:
  V_e_1/1 -> Vector Concatenate/1
  V_b_1/1 -> Vector Concatenate1/1
  V_e_2/1 -> Vector Concatenate/2
  V_b_2/1 -> Vector Concatenate1/2
  Vector Concatenate/1 -> Embedded MATLAB Function/1(Ri)
  Vector Concatenate1/1 -> Embedded MATLAB Function/2(Bi)
  a1/1 -> Mux/1
  a2/1 -> Mux/2
  Mux/1 -> Embedded MATLAB Function/3(a)
  Embedded MATLAB Function/1(q_opt) -> q_be_opt/1

== system UAVdesign_net/Utilities/Axes/Euler Rotation Matrix from Body to Earth ==
  In1 : Inport  PortDimensions=3
  Create 3x3 Matrix : UAVdesign_net/Utilities/Math/Create 3x3 Matrix  SystemSampleTime=-1
  Fcn11 : Fcn  Expr=u(5)*u(6)
  Fcn12 : Fcn  Expr=u(1)*u(2)*u(6)-u(4)*u(3)
  Fcn13 : Fcn  Expr=u(4)*u(2)*u(6)+u(1)*u(3)
  Fcn21 : Fcn  Expr=u(5)*u(3)
  Fcn22 : Fcn  Expr=u(1)*u(2)*u(3) + u(4)*u(6)
  Fcn23 : Fcn  Expr=u(4)*u(2)*u(3)-u(1)*u(6)
  Fcn31 : Fcn  Expr=-u(2)
  Fcn32 : Fcn  Expr=u(1)*u(5)
  Fcn33 : Fcn  Expr=u(4)*u(5)
  Mux : Mux  Inputs=2
  SinCos : UAVdesign_net/Utilities/Math/SinCos  SystemSampleTime=-1
  Out1 : Outport  PortDimensions=[3,3]
  wires:
  Fcn33/1 -> Create 3x3 Matrix/9
  Fcn32/1 -> Create 3x3 Matrix/8
  Fcn23/1 -> Create 3x3 Matrix/6
  Fcn22/1 -> Create 3x3 Matrix/5
  Fcn31/1 -> Create 3x3 Matrix/7
  Fcn21/1 -> Create 3x3 Matrix/4
  Fcn13/1 -> Create 3x3 Matrix/3
  Fcn12/1 -> Create 3x3 Matrix/2
  Fcn11/1 -> Create 3x3 Matrix/1
  Mux/1 -> Fcn21/1, Fcn13/1, Fcn12/1, Fcn11/1, Fcn22/1, Fcn23/1, Fcn31/1, Fcn33/1, Fcn32/1
  SinCos/2 -> Mux/2
  SinCos/1 -> Mux/1
  Create 3x3 Matrix/1 -> Out1/1
  In1/1 -> SinCos/1

== system UAVdesign_net/Utilities/Axes/Euler Rotation Matrix from Earth to Body ==
  In1 : Inport  PortDimensions=3
  Create 3x3 Matrix : UAVdesign_net/Utilities/Math/Create 3x3 Matrix  SystemSampleTime=-1
  Fcn11 : Fcn  Expr=u(5)*u(6)
  Fcn12 : Fcn  Expr=u(5)*u(3)
  Fcn13 : Fcn  Expr=-u(2)
  Fcn21 : Fcn  Expr=u(1)*u(2)*u(6) - u(4)*u(3)
  Fcn22 : Fcn  Expr=u(1)*u(2)*u(3) + u(4)*u(6)
  Fcn23 : Fcn  Expr=u(1)*u(5)
  Fcn31 : Fcn  Expr=u(4)*u(2)*u(6) + u(1)*u(3)
  Fcn32 : Fcn  Expr=u(4)*u(2)*u(3) - u(1)*u(6)
  Fcn33 : Fcn  Expr=u(4)*u(5)
  Mux : Mux  Inputs=2
  SinCos : UAVdesign_net/Utilities/Math/SinCos  SystemSampleTime=-1
  Out1 : Outport  PortDimensions=[3,3]
  wires:
  Fcn23/1 -> Create 3x3 Matrix/6
  In1/1 -> SinCos/1
  Create 3x3 Matrix/1 -> Out1/1
  SinCos/1 -> Mux/1
  SinCos/2 -> Mux/2
  Mux/1 -> Fcn32/1, Fcn33/1, Fcn31/1, Fcn23/1, Fcn22/1, Fcn11/1, Fcn12/1, Fcn13/1, Fcn21/1
  Fcn11/1 -> Create 3x3 Matrix/1
  Fcn12/1 -> Create 3x3 Matrix/2
  Fcn13/1 -> Create 3x3 Matrix/3
  Fcn21/1 -> Create 3x3 Matrix/4
  Fcn31/1 -> Create 3x3 Matrix/7
  Fcn22/1 -> Create 3x3 Matrix/5
  Fcn32/1 -> Create 3x3 Matrix/8
  Fcn33/1 -> Create 3x3 Matrix/9

== system UAVdesign_net/Utilities/Axes/Quaternions to Rotation Angles ==
  q : Inport
  Quaternion Normalize : UAVdesign_net/Utilities/Math/Quaternion Normalize  SystemSampleTime=-1
  Trigonometric Function1 : Trigonometry  Operator=atan2
  Trigonometric Function3 : Trigonometry  Operator=atan2
  Vector Concatenate : Concatenate  NumInputs=3  Mode=Vector
  fcn1 : Fcn  Expr=2*(u[3]*u[4] + u[1]*u[2])
  fcn2 : Fcn  Expr=u[1]*u[1] - u[2]*u[2] - u[3]*u[3] + u[4]*u[4]
  fcn3 : Fcn  Expr=-2*(u[2]*u[4] - u[1]*u[3])
  fcn4 : Fcn  Expr=2*(u[2]*u[3] + u[1]*u[4])
  fcn5 : Fcn  Expr=u[1]*u[1] + u[2]*u[2] - u[3]*u[3] - u[4]*u[4]
  trigFcn : Trigonometry  Operator=asin
  R1,R2,R3 : Outport
  wires:
  fcn5/1 -> Trigonometric Function3/2
  fcn4/1 -> Trigonometric Function3/1
  fcn2/1 -> Trigonometric Function1/2
  fcn1/1 -> Trigonometric Function1/1
  fcn3/1 -> trigFcn/1
  q/1 -> Quaternion Normalize/1
  Vector Concatenate/1 -> R1,R2,R3/1
  Trigonometric Function1/1 -> Vector Concatenate/1  "r1"
  trigFcn/1 -> Vector Concatenate/2  "r2"
  Trigonometric Function3/1 -> Vector Concatenate/3  "r3"
  Quaternion Normalize/1 -> fcn1/1, fcn2/1, fcn5/1, fcn4/1, fcn3/1

== system UAVdesign_net/Utilities/Axes/Rotation Angles to Quaternions ==
  "R1, R2, R3" : Inport
  1/2 : Gain  Gain=0.5  SaturateOnIntegerOverflow=on  OutDataTypeStr=Inherit: Same as input  ParamDataTypeStr=Inherit: Same as input
  Mux1 : Mux  Inputs=2
  Mux2 : Mux
  SinCos : UAVdesign_net/Utilities/Math/SinCos  SystemSampleTime=-1
  q0 : Fcn  Expr=u(4)*u(5)*u(6) + u(1)*u(2)*u(3)
  q1 : Fcn  Expr=u(1)*u(5)*u(6) - u(4)*u(2)*u(3)
  q2 : Fcn  Expr=u(4)*u(2)*u(6) + u(1)*u(5)*u(3)
  q3 : Fcn  Expr=u(4)*u(5)*u(3) - u(1)*u(2)*u(6)
  Quat : Outport  InitialOutput=0
  wires:
  q0/1 -> Mux2/1
  Mux2/1 -> Quat/1
  q3/1 -> Mux2/4
  q2/1 -> Mux2/3
  q1/1 -> Mux2/2
  Mux1/1 -> q3/1, q2/1, q1/1, q0/1
  SinCos/2 -> Mux1/2
  SinCos/1 -> Mux1/1
  1/2/1 -> SinCos/1
  "R1, R2, R3"/1 -> 1/2/1

== system UAVdesign_net/Utilities/Axes/Rotation Matrix for angular rates Body to Earth ==
  In1 : Inport  PortDimensions=3
  Create 3x3 Matrix : UAVdesign_net/Utilities/Math/Create 3x3 Matrix  SystemSampleTime=-1
  Demux : Demux  Outputs=3
  Fcn11 : Fcn  Expr=1
  Fcn12 : Fcn  Expr=u(1)*u(4)
  Fcn13 : Fcn  Expr=u(2)*u(4)
  Fcn21 : Fcn  Expr=0
  Fcn22 : Fcn  Expr=u(2)
  Fcn23 : Fcn  Expr=-u(1)
  Fcn31 : Fcn  Expr=0
  Fcn32 : Fcn  Expr=u(1)/u(3)
  Fcn33 : Fcn  Expr=u(2)/u(3)
  Mux : Mux
  Terminator : Terminator
  cosine : Trigonometry  Operator=cos
  cosine2 : Trigonometry  Operator=cos
  sine : Trigonometry
  tangent : Trigonometry  Operator=tan
  Out1 : Outport  PortDimensions=[3,3]
  wires:
  Demux/3 -> Terminator/1
  Demux/2 -> tangent/1, cosine2/1
  Demux/1 -> cosine/1, sine/1
  tangent/1 -> Mux/4
  cosine2/1 -> Mux/3
  cosine/1 -> Mux/2
  sine/1 -> Mux/1
  In1/1 -> Demux/1
  Create 3x3 Matrix/1 -> Out1/1
  Mux/1 -> Fcn32/1, Fcn33/1, Fcn31/1, Fcn23/1, Fcn22/1, Fcn11/1, Fcn12/1, Fcn13/1, Fcn21/1
  Fcn11/1 -> Create 3x3 Matrix/1
  Fcn12/1 -> Create 3x3 Matrix/2
  Fcn13/1 -> Create 3x3 Matrix/3
  Fcn21/1 -> Create 3x3 Matrix/4
  Fcn31/1 -> Create 3x3 Matrix/7
  Fcn22/1 -> Create 3x3 Matrix/5
  Fcn23/1 -> Create 3x3 Matrix/6
  Fcn32/1 -> Create 3x3 Matrix/8
  Fcn33/1 -> Create 3x3 Matrix/9

== system UAVdesign_net/Utilities/Axes/Rotation Matrix for angular rates from Earth to Body ==
  In1 : Inport  PortDimensions=3
  Create 3x3 Matrix : UAVdesign_net/Utilities/Math/Create 3x3 Matrix  SystemSampleTime=-1
  Fcn11 : Fcn  Expr=1
  Fcn12 : Fcn  Expr=0
  Fcn13 : Fcn  Expr=-u(2)
  Fcn21 : Fcn  Expr=0
  Fcn22 : Fcn  Expr=u(3)
  Fcn23 : Fcn  Expr=u(1)*u(4)
  Fcn31 : Fcn  Expr=0
  Fcn32 : Fcn  Expr=-u(1)
  Fcn33 : Fcn  Expr=u(3)*u(4)
  Mux : Mux  Inputs=2
  Selector : Selector  InputPortWidth=3  IndexOptions=Index vector (dialog)  Indices=[1 2]  OutputSizes=1
  SinCos : UAVdesign_net/Utilities/Math/SinCos  SystemSampleTime=-1
  Out1 : Outport  PortDimensions=[3,3]
  wires:
  In1/1 -> Selector/1
  Selector/1 -> SinCos/1
  Fcn33/1 -> Create 3x3 Matrix/9
  Fcn32/1 -> Create 3x3 Matrix/8
  Fcn23/1 -> Create 3x3 Matrix/6
  Fcn22/1 -> Create 3x3 Matrix/5
  Fcn31/1 -> Create 3x3 Matrix/7
  Fcn21/1 -> Create 3x3 Matrix/4
  Fcn13/1 -> Create 3x3 Matrix/3
  Fcn12/1 -> Create 3x3 Matrix/2
  Fcn11/1 -> Create 3x3 Matrix/1
  Mux/1 -> Fcn21/1, Fcn13/1, Fcn12/1, Fcn11/1, Fcn22/1, Fcn23/1, Fcn31/1, Fcn33/1, Fcn32/1
  SinCos/2 -> Mux/2
  SinCos/1 -> Mux/1
  Create 3x3 Matrix/1 -> Out1/1

== system UAVdesign_net/Utilities/Math/3x3 Cross Product ==
  A : Inport
  B : Inport  Port=2
  "A " : InportShadow  Port=1
  "B " : InportShadow  Port=2
  Subsystem : Subsystem
  Subsystem1 : Subsystem
  Sum : Sum  Inputs=+|-  SaturateOnIntegerOverflow=on  InputSameDT=on  OutDataTypeStr=Inherit: Same as first input
  C : Outport
  wires:
  Subsystem1/1(Out1) -> Sum/2
  Subsystem/1(Out1) -> Sum/1
  A/1 -> Subsystem/1(A)
  B/1 -> Subsystem/2(B)
  Sum/1 -> C/1
  "A "/1 -> Subsystem1/1(A)
  "B "/1 -> Subsystem1/2(B)

== system UAVdesign_net/Utilities/Math/Adjoint of 3x3 Matrix ==
  Matrix : Inport
  C(1,1) : Subsystem
  C(1,2) : Subsystem
  C(1,3) : Subsystem
  C(2,1) : Subsystem
  C(2,2) : Subsystem
  C(2,3) : Subsystem
  C(3,1) : Subsystem
  C(3,2) : Subsystem
  C(3,3) : Subsystem
  Create 3x3 Matrix : UAVdesign_net/Utilities/Math/Create 3x3 Matrix  SystemSampleTime=-1
  Reshape : Reshape  OutputDimensionality=Column vector (2-D)
  adj(Matrix) : Outport
  wires:
  Reshape/1 -> C(1,1)/1(Matrix), C(1,2)/1(Matrix), C(3,3)/1(Matrix), C(3,2)/1(Matrix), C(3,1)/1(Matrix), C(2,3)/1(Matrix), C(2,2)/1(Matrix), C(2,1)/1(Matrix), C(1,3)/1(Matrix)
  C(1,2)/1(C(1,2)) -> Create 3x3 Matrix/2
  C(1,3)/1(C(1,3)) -> Create 3x3 Matrix/3
  C(2,1)/1(C(2,1)) -> Create 3x3 Matrix/4
  C(2,3)/1(C(2,3)) -> Create 3x3 Matrix/6
  C(3,1)/1(C(3,1)) -> Create 3x3 Matrix/7
  C(3,2)/1(C(3,2)) -> Create 3x3 Matrix/8
  Create 3x3 Matrix/1 -> adj(Matrix)/1
  C(3,3)/1(C(3,3)) -> Create 3x3 Matrix/9
  C(2,2)/1(C(2,2)) -> Create 3x3 Matrix/5
  C(1,1)/1(C(1,1)) -> Create 3x3 Matrix/1
  Matrix/1 -> Reshape/1

== system UAVdesign_net/Utilities/Math/Create 3x3 Matrix ==
  M11 : Inport
  M12 : Inport  Port=2
  M13 : Inport  Port=3
  M21 : Inport  Port=4
  M22 : Inport  Port=5
  M23 : Inport  Port=6
  M31 : Inport  Port=7
  M32 : Inport  Port=8
  M33 : Inport  Port=9
  Mux : Mux  Inputs=9
  Reshape (9) to [3x3] column-major : Reshape  OutputDimensionality=Customize  OutputDimensions=[3,3]
  Matrix : Outport
  wires:
  Mux/1 -> Reshape (9) to [3x3] column-major/1
  M11/1 -> Mux/1
  M21/1 -> Mux/2
  M31/1 -> Mux/3
  M12/1 -> Mux/4
  M22/1 -> Mux/5
  Reshape (9) to [3x3] column-major/1 -> Matrix/1
  M32/1 -> Mux/6
  M13/1 -> Mux/7
  M23/1 -> Mux/8
  M33/1 -> Mux/9

== system UAVdesign_net/Utilities/Math/Determinant of 3x3 Matrix ==
  Matrix : Inport
  Product{,1..5} (6 alike) : Product  Inputs=1  SaturateOnIntegerOverflow=on  OutDataTypeStr=Inherit: Same as first input
  Reshape : simulink/Math Operations/Reshape  OutputDimensionality=Column vector  OutputDimensions=[1,1]
  Sum : Sum  Inputs=+--++-  SaturateOnIntegerOverflow=on
  a(1,1),a(2,2),a(3,3) : Selector  InputPortWidth=9  IndexOptions=Index vector (dialog)  Indices=[1 5 9]  OutputSizes=1
  a(1,1),a(2,3),a(3,2) : Selector  InputPortWidth=9  IndexOptions=Index vector (dialog)  Indices=[1 6 8]  OutputSizes=1
  a(1,2),a(2,1),a(3,3) : Selector  InputPortWidth=9  IndexOptions=Index vector (dialog)  Indices=[2 4 9]  OutputSizes=1
  a(1,2),a(2,3),a(3,1) : Selector  InputPortWidth=9  IndexOptions=Index vector (dialog)  Indices=[3 4 8]  OutputSizes=1
  a(1,3),a(2,1),a(3,2) : Selector  InputPortWidth=9  IndexOptions=Index vector (dialog)  Indices=[2 6 7]  OutputSizes=1
  a(1,3),a(2,2),a(3,1) : Selector  InputPortWidth=9  IndexOptions=Index vector (dialog)  Indices=[3 5 7]  OutputSizes=1
  det(Matrix) : Outport
  wires:
  Reshape/1 -> a(1,3),a(2,2),a(3,1)/1, a(1,3),a(2,1),a(3,2)/1, a(1,2),a(2,3),a(3,1)/1, a(1,2),a(2,1),a(3,3)/1, a(1,1),a(2,3),a(3,2)/1, a(1,1),a(2,2),a(3,3)/1
  Sum/1 -> det(Matrix)/1  "det(Matrix)"
  Matrix/1 -> Reshape/1
  Product5/1 -> Sum/6
  Product4/1 -> Sum/5
  Product3/1 -> Sum/4
  Product2/1 -> Sum/3
  Product1/1 -> Sum/2
  Product/1 -> Sum/1
  a(1,3),a(2,2),a(3,1)/1 -> Product5/1
  a(1,3),a(2,1),a(3,2)/1 -> Product4/1
  a(1,2),a(2,3),a(3,1)/1 -> Product3/1
  a(1,2),a(2,1),a(3,3)/1 -> Product2/1
  a(1,1),a(2,3),a(3,2)/1 -> Product1/1
  a(1,1),a(2,2),a(3,3)/1 -> Product/1

== system UAVdesign_net/Utilities/Math/Invert  3x3 Matrix ==
  Matrix : Inport
  Adjoint of 3x3 Matrix : UAVdesign_net/Utilities/Math/Adjoint of 3x3 Matrix  SystemSampleTime=-1
  Assertion : Assertion  Enabled=on  AssertionFailFcn="disp('Matrix is singular.  No matrix inverse.')"
  Determinant of 3x3 Matrix : UAVdesign_net/Utilities/Math/Determinant of 3x3 Matrix  SystemSampleTime=-1
  Product : Product  Inputs=*/  SaturateOnIntegerOverflow=on  OutDataTypeStr=Inherit: Same as first input
  Matrix' : Outport
  wires:
  Matrix/1 -> Determinant of 3x3 Matrix/1, Adjoint of 3x3 Matrix/1
  Determinant of 3x3 Matrix/1 -> Assertion/1, Product/2
  Adjoint of 3x3 Matrix/1 -> Product/1
  Product/1 -> Matrix'/1

== system UAVdesign_net/Utilities/Math/Quaternion Conjugate ==
  q : Inport
  Demux : Demux
  Gain : Gain  Gain=-1
  Gain1 : Gain  Gain=-1
  Gain2 : Gain  Gain=-1
  Mux : Mux
  q* : Outport
  wires:
  q/1 -> Demux/1
  Demux/2 -> Gain/1
  Demux/3 -> Gain1/1
  Demux/4 -> Gain2/1
  Demux/1 -> Mux/1
  Gain/1 -> Mux/2
  Gain1/1 -> Mux/3
  Gain2/1 -> Mux/4
  Mux/1 -> q*/1

== system UAVdesign_net/Utilities/Math/Quaternion Derivative ==
  p q r : Inport
  q0 q1 q2 q3 : Inport  Port=2
  Constant : Constant
  Dot Product : DotProduct  OutDataTypeStr=Inherit: Inherit via internal rule
  High Gain Quaternion Normalization : Gain  Gain=k_quat  SaturateOnIntegerOverflow=on  OutDataTypeStr=Inherit: Same as input  ParamDataTypeStr=Inherit: Same as input
  Mux1 : Mux  Inputs=[3 4 1]
  Mux2 : Mux
  Sum : Sum  Inputs=|+-  SaturateOnIntegerOverflow=on  InputSameDT=on  OutDataTypeStr=Inherit: Same as first input
  q0dot : Fcn  Expr=-0.5 * ( u[5]*u[1]+u[6]*u[2]+u[7]*u[3] ) + u[8]*u[4]
  q1dot : Fcn  Expr=0.5 * ( u[4]*u[1]+u[6]*u[3]-u[7]*u[2] ) + u[8]*u[5]
  q2dot : Fcn  Expr=0.5 * ( u[4]*u[2]+u[7]*u[1]-u[5]*u[3] ) + u[8]*u[6]
  q3dot : Fcn  Expr=0.5 * ( u[4]*u[3]+u[5]*u[2]-u[6]*u[1] ) + u[8]*u[7]
  qdot : Outport  InitialOutput=0
  wires:
  p q r/1 -> Mux1/1
  Dot Product/1 -> Sum/2
  High Gain Quaternion Normalization/1 -> Mux1/3
  Sum/1 -> High Gain Quaternion Normalization/1
  Constant/1 -> Sum/1
  Mux2/1 -> qdot/1
  q0dot/1 -> Mux2/1
  q1dot/1 -> Mux2/2
  q2dot/1 -> Mux2/3
  Mux1/1 -> q2dot/1, q3dot/1, q0dot/1, q1dot/1
  q3dot/1 -> Mux2/4
  q0 q1 q2 q3/1 -> Dot Product/1, Dot Product/2, Mux1/2

== system UAVdesign_net/Utilities/Math/Quaternion Division ==
  q : Inport
  r : Inport  Port=2
  Mux1 : Mux
  Product{1..4} (4 alike) : Product  Inputs=*/  RndMeth=Zero
  Quaternion Norm : UAVdesign_net/Utilities/Math/Quaternion Norm  SystemSampleTime=-1
  q0 : Subsystem
  q1 : Subsystem
  q2 : Subsystem
  q3 : Subsystem
  q/r : Outport
  wires:
  Mux1/1 -> q/r/1
  Product4/1 -> Mux1/3
  Product2/1 -> Mux1/2
  Product1/1 -> Mux1/1
  q/1 -> q3/1(q), q2/1(q), q1/1(q), q0/1(q)
  r/1 -> q2/2(r), Quaternion Norm/1, q3/2(r), q1/2(r), q0/2(r)
  q0/1(q0) -> Product1/1
  q1/1(q1) -> Product2/1
  q2/1(q2) -> Product4/1
  q3/1(q3) -> Product3/1
  Product3/1 -> Mux1/4
  Quaternion Norm/1 -> Product1/2, Product2/2, Product4/2, Product3/2

== system UAVdesign_net/Utilities/Math/Quaternion Inverse ==
  q : Inport
  Demux : Demux
  Divide{,1..3} (4 alike) : Product  Inputs=*/
  Mux : Mux
  Quaternion Conjugate : UAVdesign_net/Utilities/Math/Quaternion Conjugate  SystemSampleTime=-1
  Quaternion Norm : UAVdesign_net/Utilities/Math/Quaternion Norm  SystemSampleTime=-1
  Inv(q) : Outport
  wires:
  Demux/2 -> Divide1/1
  Demux/3 -> Divide2/1
  Demux/4 -> Divide3/1
  Divide3/1 -> Mux/4
  Divide2/1 -> Mux/3
  Divide1/1 -> Mux/2
  Mux/1 -> Inv(q)/1
  Demux/1 -> Divide/1
  Quaternion Conjugate/1 -> Demux/1
  Quaternion Norm/1 -> Divide2/2, Divide3/2, Divide1/2, Divide/2
  q/1 -> Quaternion Norm/1, Quaternion Conjugate/1
  Divide/1 -> Mux/1

== system UAVdesign_net/Utilities/Math/Quaternion Minimum Rotation ==
  q : Inport
  Gain : Gain  Gain=-1
  Selector : Selector  InputPortWidth=4  IndexOptions=Index vector (dialog)  Indices=[1]  OutputSizes=1
  Switch : Switch
  min(q) : Outport
  wires:
  Gain/1 -> Switch/3
  Selector/1 -> Switch/2
  q/1 -> Gain/1, Switch/1, Selector/1
  Switch/1 -> min(q)/1
